simulink model "sistema_completo_discreto_codificado"  (R2023a)
settings: Solver=VariableStepAuto  StartTime=0.0  StopTime=15  MaxStep=1e-3  RelTol=1e-3
values from neighbouring files (symbols this model uses):
  alpha_Cu = 3.9e-3    (= 0.0039)    [variables.m]
  b_a = J_eq * (2*zeta + 1) * omega_pos    [Polos_con_Jeq.m]
  b_eq = b_eq_max    [FrecuenciaNatural_Amortiguamiento.m]    (also in variables.m = 2.19444444444e-05)
  C_ts = 0.818    [variables.m]
  J_eq = J_eq_max    [FrecuenciaNatural_Amortiguamiento.m]    (also in variables.m = 4.58263888889e-05)
  k_l = m*l_cm + m_l*l_l    (= 1)    [variables.m]
  K_sa = J_eq * (2*zeta + 1) * omega_pos^2    [Polos_con_Jeq.m]
  K_sia = J_eq * omega_pos^3    [Polos_con_Jeq.m]
  L_d = 6.6e-3    (= 0.0066)    [variables.m]
  L_ls = 0.8e-3    (= 0.0008)    [variables.m]
  L_q = 5.8e-3    (= 0.0058)    [variables.m]
  lambda_m = 0.016    [variables.m]
  Pp = 3    [variables.m]
  r = 120    [esp_de_operacion.m]    (also in variables.m)
  R_ts = 146.7    [variables.m]
  T_s_ref = 20    [Polos_ceros_Rs.m]
undefined symbols (not defined in the file or in its folder): k_i, k_omega2, k_theta2, omega_n_i, omega_n_pos, omega_n_v, R_s_ref, tau, Ts, Vsl_max, zitta
libraries: SignalEditorBlockLib x5
settings Model: Creator=juanf  LastModifiedBy=Juan

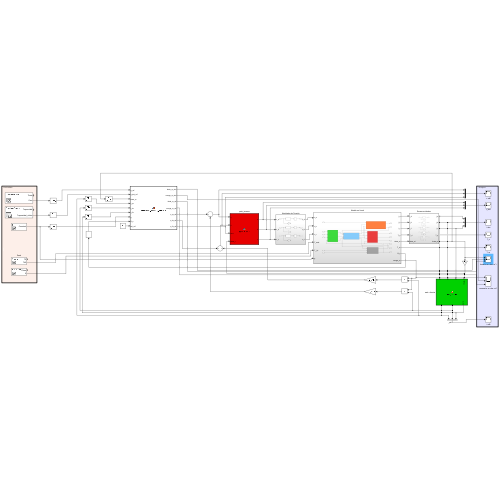
[thumbnail: Simulink's stored preview of the top-level diagram]
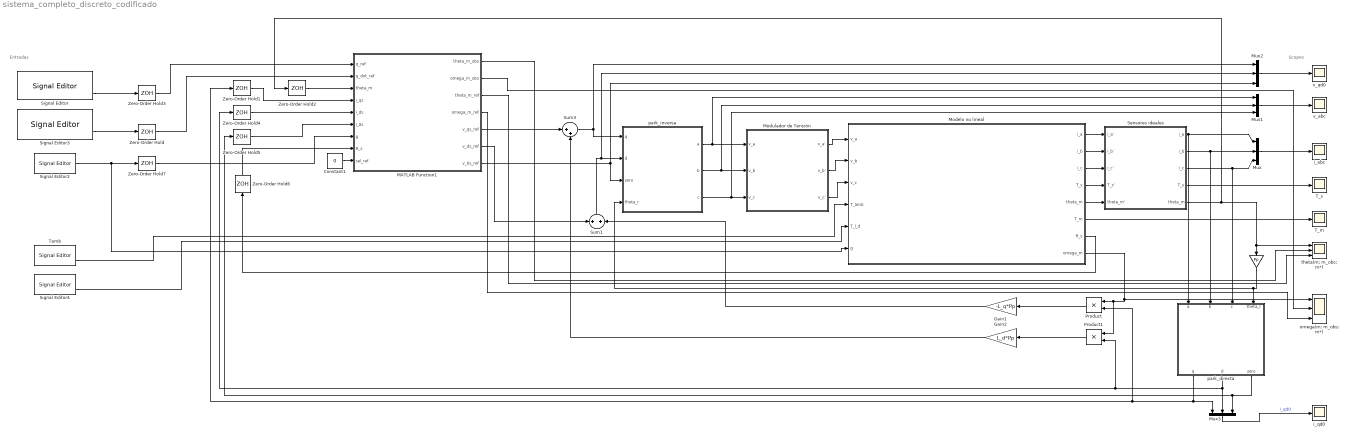
== system sistema_completo_discreto_codificado ==
  note: Scopes
  note: Entradas
  " " : Gain  Gain=Pp
  Constant1 : Constant  Value=0
  Gain1 : Gain  Gain=-L_q*Pp
  Gain2 : Gain  Gain=L_d*Pp
  MATLAB Function1 : MATLAB Function  TreatAsAtomicUnit=on
  Modelo no lineal : Subsystem
  Modulador de Tensión : Subsystem
  Mux{,1..3} (4 alike) : Mux  Inputs=3
  Product : Product
  Product1 : Product
  Sensores ideales : Subsystem
  Signal Editor : SignalEditorBlockLib/Signal Editor  FileName=Consigna_Theta.mat  ActiveScenario=ConsignaTheta  ActiveSignal=Theta  IsBus=off  OutputBusObjectStr=Bus: BusObject  SampleTime=0  ZeroCross=off  OutputAfterFinalValue=Setting to zero  Unit=inherit  PreserveSignalName=on  ApplySigPropsToAllScenarios=on
  Signal Editor2 : SignalEditorBlockLib/Signal Editor  FileName=D:\Facultad\AyME\Automatica-y-maquinas-electricas-final\Matlab - Simulink\señales\g.mat  ActiveScenario=g  ActiveSignal=Constant  IsBus=off  OutputBusObjectStr=Bus: BusObject  SampleTime=0  Interpolate=off  ZeroCross=off  OutputAfterFinalValue=Setting to zero  Unit=inherit  PreserveSignalName=on  ApplySigPropsToAllScenarios=on
  Signal Editor3 : SignalEditorBlockLib/Signal Editor  FileName=D:\Facultad\AyME\Automatica-y-maquinas-electricas-final\Matlab - Simulink\señales\señal_omega_suave.mat  ActiveScenario=ConsignaOmega  ActiveSignal=Trapezoidal  IsBus=off  OutputBusObjectStr=Bus: BusObject  SampleTime=0  Interpolate=off  ZeroCross=off  OutputAfterFinalValue=Setting to zero  Unit=inherit  PreserveSignalName=on  ApplySigPropsToAllScenarios=on
  Signal Editor4 : SignalEditorBlockLib/Signal Editor  FileName=D:\Facultad\AyME\Automatica-y-maquinas-electricas-final\Matlab - Simulink\señales\senal_Tld.mat  ActiveScenario=Senal_Tld  ActiveSignal=Pulse  IsBus=off  OutputBusObjectStr=Bus: BusObject  SampleTime=0  Interpolate=off  ZeroCross=off  OutputAfterFinalValue=Setting to zero  Unit=inherit  PreserveSignalName=on  ApplySigPropsToAllScenarios=on
  Sum1 : Sum  Inputs=+|+
  Sum3 : Sum  Inputs=|++
  T_m : Scope
  T_s : Scope
  Tamb : SignalEditorBlockLib/Signal Editor  FileName=D:\Facultad\AyME\Automatica-y-maquinas-electricas-final\Matlab - Simulink\señales\senal_Tamb.mat  ActiveScenario=T_amb  ActiveSignal=T0  IsBus=off  OutputBusObjectStr=Bus: BusObject  SampleTime=0  Interpolate=off  ZeroCross=off  OutputAfterFinalValue=Setting to zero  Unit=inherit  PreserveSignalName=on  ApplySigPropsToAllScenarios=on
  Zero-Order Hold{,1..7} (8 alike) : ZeroOrderHold  SampleTime=Ts
  i_abc : Scope
  i_qd0 : Scope
  omega(m; m_obs; m*) : Scope  NumInputPorts=3
  park_directa : MATLAB Function  TreatAsAtomicUnit=on
  park_inversa : MATLAB Function  TreatAsAtomicUnit=on
  theta(m; m_obs; m*) : Scope  NumInputPorts=3
  v_abc : Scope
  v_qd0 : Scope
  wires:
  park_inversa/1(a) -> Mux1/1, Modulador de Tensión/1(v_a)
  park_inversa/2(b) -> Mux1/2, Modulador de Tensión/2(v_b)
  park_inversa/3(c) -> Mux1/3, Modulador de Tensión/3(v_c)
  Modulador de Tensión/1(v_a') -> Modelo no lineal/1(v_a)
  Modulador de Tensión/2(v_b') -> Modelo no lineal/2(v_b)
  Modulador de Tensión/3(v_c') -> Modelo no lineal/3(v_c)
  Modelo no lineal/1(i_a) -> Sensores ideales/1(i_a')
  Modelo no lineal/2(i_b) -> Sensores ideales/2(i_b')
  Modelo no lineal/3(i_c) -> Sensores ideales/3(i_c')
  Modelo no lineal/4(T_s) -> Sensores ideales/4(T_s')
  Modelo no lineal/5(theta_m) -> Sensores ideales/5(theta_m')
  Modelo no lineal/6(T_m) -> T_m/1
  Sensores ideales/1(i_a) -> Mux/1, park_directa/1(a)
  Sensores ideales/2(i_b) -> Mux/2, park_directa/2(b)
  Sensores ideales/3(i_c) -> Mux/3, park_directa/3(c)
  Modelo no lineal/8(omega_m) -> Product1/1, Product/1, omega(m; m_obs; m*)/1
  Sum3/1 -> park_inversa/1(q), Mux2/1
  Sensores ideales/4(T_s) -> T_s/1
  park_directa/1(q) -> Product/2, Zero-Order Hold1/1, Mux3/1
  park_directa/2(d) -> Mux3/2, Zero-Order Hold4/1, Product1/2
  park_directa/3(zero) -> Mux3/3, Zero-Order Hold5/1
  " "/1 -> park_inversa/4(theta_r), park_directa/4(theta_r)
  Product/1 -> Gain1/1
  Mux/1 -> i_abc/1
  Mux1/1 -> v_abc/1
  Mux2/1 -> v_qd0/1
  Mux3/1 -> i_qd0/1  "i_qd0"
  Sum1/1 -> Mux2/2, park_inversa/2(d)
  Product1/1 -> Gain2/1
  Gain2/1 -> Sum3/2
  Gain1/1 -> Sum1/2
  Signal Editor2/1 -> Zero-Order Hold7/1, Modelo no lineal/6(g)
  Tamb/2 -> Modelo no lineal/4(T_amb)
  Modelo no lineal/7(R_s) -> Zero-Order Hold6/1
  Signal Editor4/2 -> Modelo no lineal/5(T_l_d)
  Zero-Order Hold/1 -> MATLAB Function1/2(q_dot_ref)
  Zero-Order Hold3/1 -> MATLAB Function1/1(q_ref)
  Signal Editor/2 -> Zero-Order Hold3/1
  Sensores ideales/5(theta_m) -> " "/1, theta(m; m_obs; m*)/1, Zero-Order Hold2/1
  Constant1/1 -> MATLAB Function1/9(sel_ref)
  MATLAB Function1/5(v_qs_ref) -> Sum3/1
  MATLAB Function1/7(v_0s_ref) -> Mux2/3, park_inversa/3(zero)
  MATLAB Function1/6(v_ds_ref) -> Sum1/1
  Zero-Order Hold1/1 -> MATLAB Function1/4(i_qs)
  Zero-Order Hold4/1 -> MATLAB Function1/5(i_ds)
  Zero-Order Hold5/1 -> MATLAB Function1/6(i_0s)
  Zero-Order Hold6/1 -> MATLAB Function1/8(R_s)
  Zero-Order Hold7/1 -> MATLAB Function1/7(g)
  MATLAB Function1/1(theta_m_obs) -> theta(m; m_obs; m*)/2
  MATLAB Function1/3(theta_m_ref) -> theta(m; m_obs; m*)/3
  MATLAB Function1/2(omega_m_obs) -> omega(m; m_obs; m*)/2
  MATLAB Function1/4(omega_m_ref) -> omega(m; m_obs; m*)/3
  Zero-Order Hold2/1 -> MATLAB Function1/3(theta_m)
  Signal Editor3/2 -> Zero-Order Hold/1

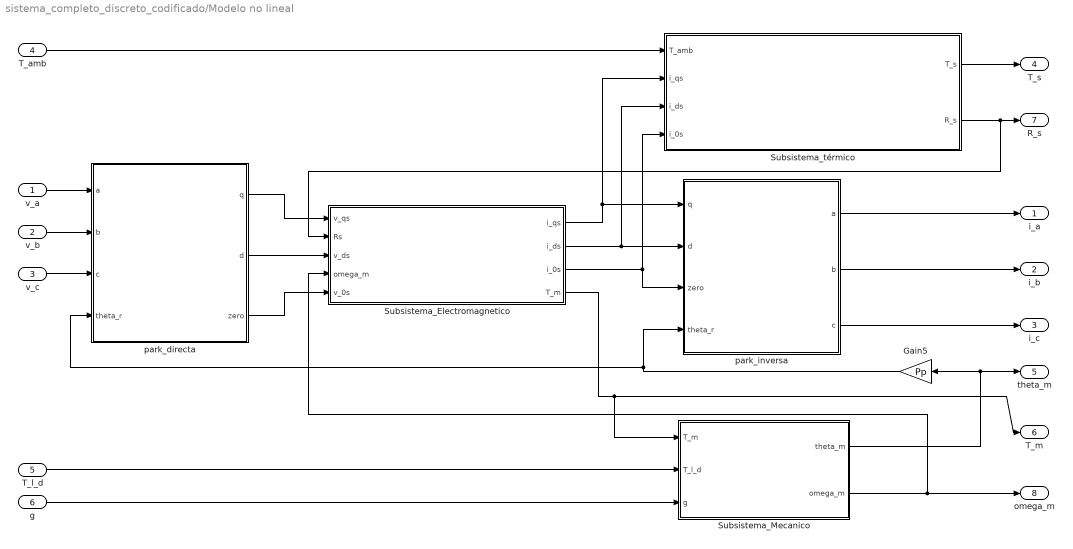
== system sistema_completo_discreto_codificado/Modelo no lineal ==
  v_a : Inport
  v_b : Inport  Port=2
  v_c : Inport  Port=3
  T_amb : Inport  Port=4
  T_l_d : Inport  Port=5
  g : Inport  Port=6
  Gain5 : Gain  Gain=Pp
  Subsistema_Electromagnetico : Subsystem
  Subsistema_Mecanico : Subsystem
  Subsistema_térmico : Subsystem
  park_directa : MATLAB Function  TreatAsAtomicUnit=on
  park_inversa : MATLAB Function  TreatAsAtomicUnit=on
  i_a : Outport
  i_b : Outport  Port=2
  i_c : Outport  Port=3
  T_s : Outport  Port=4
  theta_m : Outport  Port=5
  T_m : Outport  Port=6
  R_s : Outport  Port=7
  omega_m : Outport  Port=8
  wires:
  v_b/1 -> park_directa/2(b)
  Subsistema_Mecanico/1(theta_m) -> theta_m/1, Gain5/1
  T_l_d/1 -> Subsistema_Mecanico/2(T_l_d)
  park_directa/2(d) -> Subsistema_Electromagnetico/3(v_ds)
  Subsistema_Electromagnetico/4(T_m) -> Subsistema_Mecanico/1(T_m), T_m/1
  T_amb/1 -> Subsistema_térmico/1(T_amb)
  Subsistema_térmico/1(T_s) -> T_s/1
  Gain5/1 -> park_directa/4(theta_r), park_inversa/4(theta_r)
  v_a/1 -> park_directa/1(a)
  Subsistema_Mecanico/2(omega_m) -> omega_m/1, Subsistema_Electromagnetico/4(omega_m)
  park_directa/1(q) -> Subsistema_Electromagnetico/1(v_qs)
  Subsistema_térmico/2(R_s) -> Subsistema_Electromagnetico/2(Rs), R_s/1
  v_c/1 -> park_directa/3(c)
  park_inversa/2(b) -> i_b/1
  Subsistema_Electromagnetico/2(i_ds) -> park_inversa/2(d), Subsistema_térmico/3(i_ds)
  park_inversa/1(a) -> i_a/1
  Subsistema_Electromagnetico/1(i_qs) -> park_inversa/1(q), Subsistema_térmico/2(i_qs)
  park_inversa/3(c) -> i_c/1
  Subsistema_Electromagnetico/3(i_0s) -> park_inversa/3(zero), Subsistema_térmico/4(i_0s)
  park_directa/3(zero) -> Subsistema_Electromagnetico/5(v_0s)
  g/1 -> Subsistema_Mecanico/3(g)

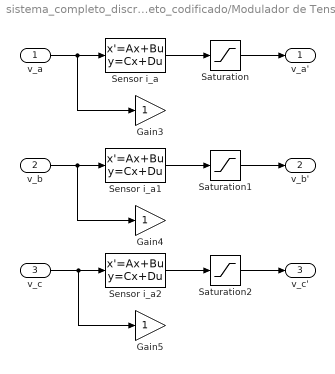
== system sistema_completo_discreto_codificado/Modulador de Tensión ==
  v_a : Inport
  v_b : Inport  Port=2
  v_c : Inport  Port=3
  Gain3 : Gain
  Gain4 : Gain
  Gain5 : Gain
  Saturation : Saturate  UpperLimit=Vsl_max  LowerLimit=-Vsl_max
  Saturation1 : Saturate  UpperLimit=Vsl_max  LowerLimit=-Vsl_max
  Saturation2 : Saturate  UpperLimit=Vsl_max  LowerLimit=-Vsl_max
  Sensor i_a : StateSpace  A=[0 1 ; -omega_n_v^2 -2*zitta*omega_n_v]  B=[0; omega_n_v^2]  C=[1 0]  D=[0]  InitialCondition=0  AllowTunableDMatrix=on
  Sensor i_a1 : StateSpace  A=[0 1 ; -omega_n_v^2 -2*zitta*omega_n_v]  B=[0; omega_n_v^2]  C=[1 0]  D=[0]  InitialCondition=0  AllowTunableDMatrix=on
  Sensor i_a2 : StateSpace  A=[0 1 ; -omega_n_v^2 -2*zitta*omega_n_v]  B=[0; omega_n_v^2]  C=[1 0]  D=[0]  InitialCondition=0  AllowTunableDMatrix=on
  v_a' : Outport
  v_b' : Outport  Port=2
  v_c' : Outport  Port=3
  wires:
  v_b/1 -> Sensor i_a1/1, Gain4/1
  v_a/1 -> Gain3/1, Sensor i_a/1
  Sensor i_a1/1 -> Saturation1/1
  Sensor i_a2/1 -> Saturation2/1
  v_c/1 -> Sensor i_a2/1, Gain5/1
  Sensor i_a/1 -> Saturation/1
  Saturation/1 -> v_a'/1
  Saturation1/1 -> v_b'/1
  Saturation2/1 -> v_c'/1

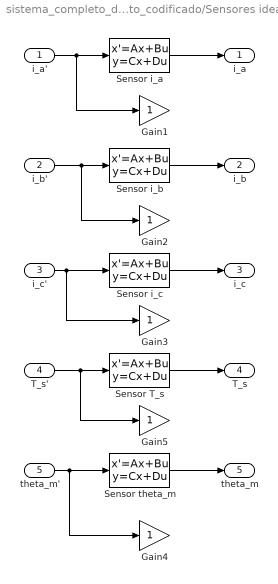
== system sistema_completo_discreto_codificado/Sensores ideales ==
  i_a' : Inport
  i_b' : Inport  Port=2
  i_c' : Inport  Port=3
  T_s' : Inport  Port=4
  theta_m' : Inport  Port=5
  Gain{1..5} (5 alike) : Gain
  Sensor T_s : StateSpace  A=[-1/tau]  B=[1/tau]  C=[1]  D=[0]  InitialCondition=40  AllowTunableDMatrix=on
  Sensor i_a : StateSpace  A=[0 1 ; -omega_n_i^2 -2*zitta*omega_n_i]  B=[0; omega_n_i^2]  C=[1 0]  D=[0]  InitialCondition=0  AllowTunableDMatrix=on
  Sensor i_b : StateSpace  A=[0 1 ; -omega_n_i^2 -2*zitta*omega_n_i]  B=[0; omega_n_i^2]  C=[1 0]  D=[0]  InitialCondition=0  AllowTunableDMatrix=on
  Sensor i_c : StateSpace  A=[0 1 ; -omega_n_i^2 -2*zitta*omega_n_i]  B=[0; omega_n_i^2]  C=[1 0]  D=[0]  InitialCondition=0  AllowTunableDMatrix=on
  Sensor theta_m : StateSpace  A=[0 1 ; -omega_n_pos^2 -2*zitta*omega_n_pos]  B=[0; omega_n_pos^2]  C=[1 0]  D=[0]  InitialCondition=0  AllowTunableDMatrix=on
  i_a : Outport
  i_b : Outport  Port=2
  i_c : Outport  Port=3
  T_s : Outport  Port=4
  theta_m : Outport  Port=5
  wires:
  i_a'/1 -> Gain1/1, Sensor i_a/1
  i_b'/1 -> Gain2/1, Sensor i_b/1
  i_c'/1 -> Gain3/1, Sensor i_c/1
  T_s'/1 -> Gain5/1, Sensor T_s/1
  theta_m'/1 -> Gain4/1, Sensor theta_m/1
  Sensor theta_m/1 -> theta_m/1
  Sensor T_s/1 -> T_s/1
  Sensor i_c/1 -> i_c/1
  Sensor i_b/1 -> i_b/1
  Sensor i_a/1 -> i_a/1

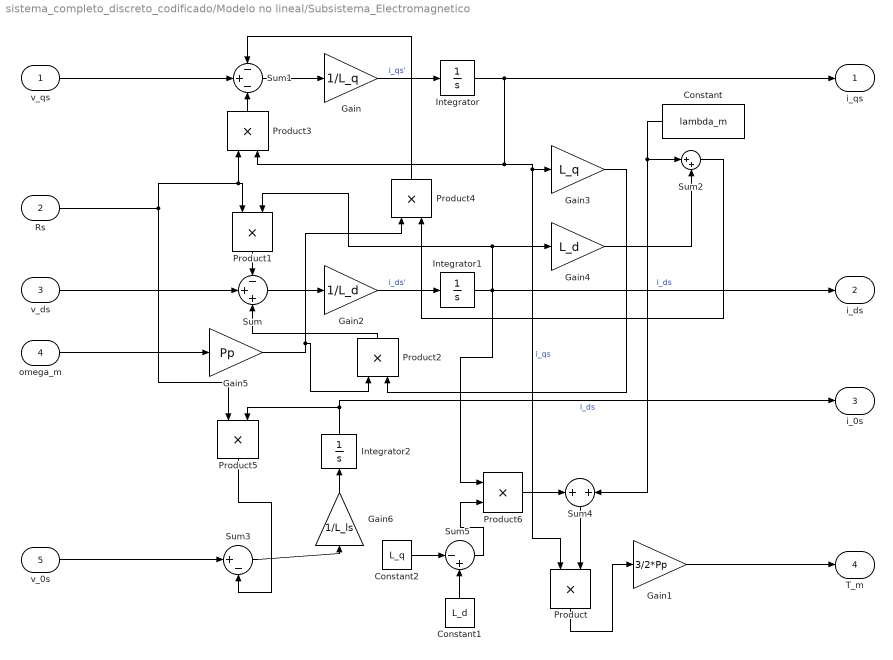
== system sistema_completo_discreto_codificado/Modelo no lineal/Subsistema_Electromagnetico ==
  v_qs : Inport
  Rs : Inport  Port=2
  v_ds : Inport  Port=3
  omega_m : Inport  Port=4
  v_0s : Inport  Port=5
  Constant : Constant  Value=lambda_m
  Constant1 : Constant  Value=L_d
  Constant2 : Constant  Value=L_q
  Gain : Gain  Gain=1/L_q
  Gain1 : Gain  Gain=3/2*Pp
  Gain2 : Gain  Gain=1/L_d
  Gain3 : Gain  Gain=L_q
  Gain4 : Gain  Gain=L_d
  Gain5 : Gain  Gain=Pp
  Gain6 : Gain  Gain=1/L_ls
  Integrator : Integrator
  Integrator1 : Integrator
  Integrator2 : Integrator
  Product{,1..6} (7 alike) : Product
  Sum : Sum  Inputs=-++
  Sum1 : Sum  Inputs=-+-
  Sum2 : Sum  Inputs=|++
  Sum3 : Sum  Inputs=|+-
  Sum4 : Sum
  Sum5 : Sum  Inputs=|-+
  i_qs : Outport
  i_ds : Outport  Port=2
  i_0s : Outport  Port=3
  T_m : Outport  Port=4
  wires:
  Gain1/1 -> T_m/1
  Product/1 -> Gain1/1
  v_qs/1 -> Sum1/2
  Sum1/1 -> Gain/1
  Gain/1 -> Integrator/1  "i_qs'"
  Integrator/1 -> Product/1, Gain3/1, Product3/2, i_qs/1  "i_qs"
  Product3/1 -> Sum1/3
  Rs/1 -> Product3/1, Product1/1, Product5/1
  Product4/1 -> Sum1/1
  Product1/1 -> Sum/1
  v_ds/1 -> Sum/2
  Sum/1 -> Gain2/1
  Gain2/1 -> Integrator1/1  "i_ds'"
  Integrator1/1 -> i_ds/1, Product6/1, Gain4/1, Product1/2  "i_ds"
  Constant/1 -> Sum4/2, Sum2/1
  Sum2/1 -> Product4/2
  omega_m/1 -> Gain5/1
  Gain5/1 -> Product2/1, Product4/1
  Product2/1 -> Sum/3
  Gain4/1 -> Sum2/2
  Gain3/1 -> Product2/2
  v_0s/1 -> Sum3/1
  Product5/1 -> Sum3/2
  Sum3/1 -> Gain6/1
  Gain6/1 -> Integrator2/1
  Integrator2/1 -> Product5/2, i_0s/1  "i_ds"
  Constant1/1 -> Sum5/2
  Constant2/1 -> Sum5/1
  Product6/1 -> Sum4/1
  Sum5/1 -> Product6/2
  Sum4/1 -> Product/2

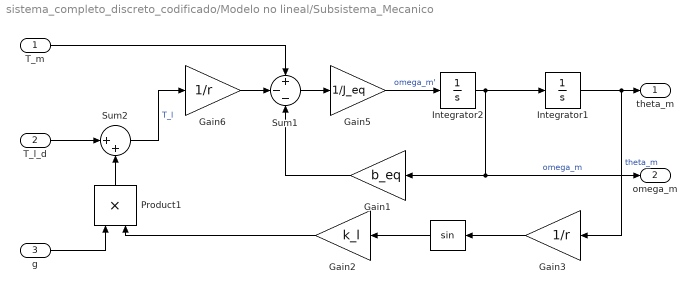
== system sistema_completo_discreto_codificado/Modelo no lineal/Subsistema_Mecanico ==
  T_m : Inport
  T_l_d : Inport  Port=2
  g : Inport  Port=3
  " " : Trigonometry
  Gain1 : Gain  Gain=b_eq
  Gain2 : Gain  Gain=k_l
  Gain3 : Gain  Gain=1/r
  Gain5 : Gain  Gain=1/J_eq
  Gain6 : Gain  Gain=1/r
  Integrator1 : Integrator
  Integrator2 : Integrator
  Product1 : Product
  Sum1 : Sum  Inputs=+--
  Sum2 : Sum  Inputs=|++
  theta_m : Outport
  omega_m : Outport  Port=2
  wires:
  Product1/1 -> Sum2/2
  T_l_d/1 -> Sum2/1
  Integrator1/1 -> Gain3/1, theta_m/1  "theta_m"
  Gain3/1 -> " "/1
  " "/1 -> Gain2/1
  Gain1/1 -> Sum1/3
  Sum1/1 -> Gain5/1
  Sum2/1 -> Gain6/1  "T_l"
  Gain6/1 -> Sum1/2
  Integrator2/1 -> Integrator1/1, Gain1/1, omega_m/1  "omega_m"
  Gain5/1 -> Integrator2/1  "omega_m'"
  Gain2/1 -> Product1/2
  T_m/1 -> Sum1/1
  g/1 -> Product1/1

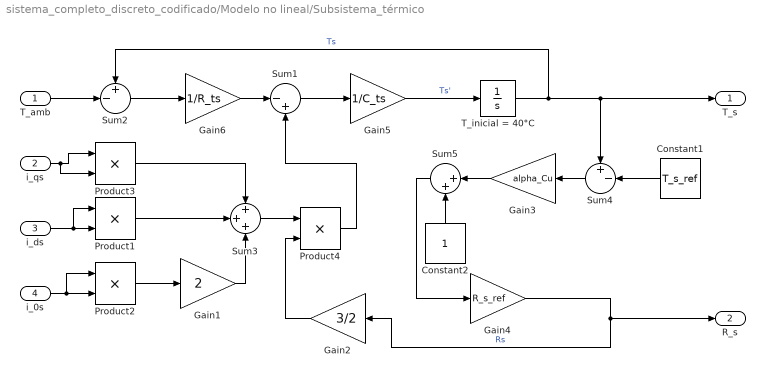
== system sistema_completo_discreto_codificado/Modelo no lineal/Subsistema_térmico ==
  T_amb : Inport
  i_qs : Inport  Port=2
  i_ds : Inport  Port=3
  i_0s : Inport  Port=4
  Constant1 : Constant  Value=T_s_ref
  Constant2 : Constant
  Gain1 : Gain  Gain=2
  Gain2 : Gain  Gain=3/2
  Gain3 : Gain  Gain=alpha_Cu
  Gain4 : Gain  Gain=R_s_ref
  Gain5 : Gain  Gain=1/C_ts
  Gain6 : Gain  Gain=1/R_ts
  Product{1..4} (4 alike) : Product
  Sum1 : Sum  Inputs=|-+
  Sum2 : Sum  Inputs=+-|
  Sum3 : Sum  Inputs=+++
  Sum4 : Sum  Inputs=+-|
  Sum5 : Sum  Inputs=|++
  T_inicial = 40°C : Integrator  InitialCondition=40
  T_s : Outport
  R_s : Outport  Port=2
  wires:
  Gain5/1 -> T_inicial = 40°C/1  "Ts'"
  Sum1/1 -> Gain5/1
  Sum2/1 -> Gain6/1
  T_amb/1 -> Sum2/2
  T_inicial = 40°C/1 -> Sum4/1, T_s/1, Sum2/1  "Ts"
  i_qs/1 -> Product3/2, Product3/1
  i_0s/1 -> Product2/1, Product2/2
  Product2/1 -> Gain1/1
  Gain1/1 -> Sum3/3
  Product1/1 -> Sum3/2
  Product3/1 -> Sum3/1
  Sum3/1 -> Product4/1
  Gain2/1 -> Product4/2
  Gain6/1 -> Sum1/1
  Product4/1 -> Sum1/2
  Constant1/1 -> Sum4/2
  Sum4/1 -> Gain3/1
  Constant2/1 -> Sum5/2
  Sum5/1 -> Gain4/1
  Gain4/1 -> Gain2/1, R_s/1  "Rs"
  Gain3/1 -> Sum5/1
  i_ds/1 -> Product1/2, Product1/1

== matlab function sistema_completo_discreto_codificado/MATLAB Function1 ==
  data: q_ref input; q_dot_ref input; theta_m input; i_qs input; i_ds input; i_0s input; g input; R_s input; Ts parameter; r parameter; J_eq parameter; b_a parameter; K_sa parameter; K_sia parameter; k_i parameter; k_theta2 parameter; theta_m_obs output; omega_m_obs output; k_omega2 parameter; b_eq parameter; k_l parameter; Pp parameter; lambda_m parameter; L_d parameter; L_q parameter; L_ls parameter; theta_m_ref output; omega_m_ref output; sel_ref input; v_qs_ref output; v_ds_ref output; v_0s_ref output
function [theta_m_obs, omega_m_obs, theta_m_ref, omega_m_ref, ...
          v_qs_ref, v_ds_ref, v_0s_ref] = controlador_discreto_completo( ...
          q_ref, q_dot_ref, theta_m, i_qs, i_ds, i_0s, g, R_s, ...
          Ts, r, J_eq, b_a, K_sa, K_sia, k_i, k_theta2, k_omega2, ...
          b_eq, k_l, Pp, lambda_m, L_d, L_q, L_ls, sel_ref)
%CONTROLADOR_DISCRETO_COMPLETO
% Reemplaza en una sola MATLAB Function todos los bloques externos a la
% planta del modelo discreto:
%   1) Setpoint
%   2) PID externo
%   3) Observador
%   4) Modulador de torque
%   5) Modulador de corriente
%   6) Desacople electromagnetico
%
% Para que reemplace tambien a los Zero-Order Hold del esquema, el bloque
% MATLAB Function debe ejecutarse con tiempo de muestreo Ts.

persistent initialized

persistent C_halfTs C_invJeq C_invTs
persistent C_r C_inv_r
persistent C_ba C_Ksa C_Ksia
persistent C_ktheta2 C_komega2 C_ki
persistent C_beq C_kg_over_r C_three_halves_pp
persistent C_lambda_m C_Ld C_Lq C_Lls
persistent C_Ld_minus_Lq
persistent C_kiq C_kid C_ki0

% Memorias para generacion de referencias
persistent ref_theta_prev
persistent ref_omega_u_prev ref_omega_y_prev

% PID externo
persistent pid_u1_prev pid_y1_prev
persistent pid_u2_prev pid_y2_prev

% Observador
persistent obs_z_eps obs_z_alpha obs_z_thetadot
persistent obs_xi_u_prev obs_xi_y_prev
persistent obs_omega_u_prev obs_omega_y_prev
persistent obs_theta_u_prev obs_theta_y_prev

if isempty(initialized)
    initialized = true;

    C_halfTs = Ts / 2;
    C_invJeq = 1 / J_eq;
    C_invTs  = 1 / Ts;

    C_r     = r;
    C_inv_r = 1 / r;

    C_ba    = b_a;
    C_Ksa   = K_sa;
    C_Ksia  = K_sia;

    C_ktheta2 = k_theta2;
    C_komega2 = k_omega2;
    C_ki      = k_i;

    C_beq             = b_eq;
    C_kg_over_r       = k_l / r;
    C_three_halves_pp = 1.5 * Pp;

    C_lambda_m    = lambda_m;
    C_Ld          = L_d;
    C_Lq          = L_q;
    C_Lls         = L_ls;
    C_Ld_minus_Lq = L_d - L_q;

    C_kiq = 5000 * L_q;
    C_kid = 5000 * L_d;
    C_ki0 = 5000 * L_ls;

    ref_theta_prev   = 0;
    ref_omega_u_prev = 0;
    ref_omega_y_prev = 0;

    pid_u1_prev = 0;
    pid_y1_prev = 0;
    pid_u2_prev = 0;
    pid_y2_prev = 0;

    obs_z_eps      = 0;
    obs_z_alpha    = 0;
    obs_z_thetadot = 0;

    obs_xi_u_prev    = 0;
    obs_xi_y_prev    = 0;
    obs_omega_u_prev = 0;
    obs_omega_y_prev = 0;
    obs_theta_u_prev = 0;
    obs_theta_y_prev = 0;
end

% =========================================================================
% A) OBSERVADOR: SALIDAS ESTIMADAS
% =========================================================================
[x_I, obs_xi_u_prev, obs_xi_y_prev] = ...
    f_tustin(obs_z_eps, obs_xi_u_prev, obs_xi_y_prev, C_halfTs);

[omega_m_obs, obs_omega_u_prev, obs_omega_y_prev] = ...
    f_tustin(obs_z_alpha, obs_omega_u_prev, obs_omega_y_prev, C_halfTs);

[theta_m_obs, obs_theta_u_prev, obs_theta_y_prev] = ...
    f_tustin(obs_z_thetadot, obs_theta_u_prev, obs_theta_y_prev, C_halfTs);

% =========================================================================
% B) GENERACION DE REFERENCIAS
% sel_ref = 0 -> referencia principal de velocidad
% sel_ref = 1 -> referencia principal de posicion
% =========================================================================
if sel_ref == 0
    omega_m_ref = C_r * q_dot_ref;

    [theta_m_ref, ref_omega_u_prev, ref_omega_y_prev] = ...
        f_tustin(omega_m_ref, ref_omega_u_prev, ref_omega_y_prev, C_halfTs);

    ref_theta_prev = theta_m_ref;
else
    theta_m_ref = C_r * q_ref;
    omega_m_ref = (theta_m_ref - ref_theta_prev) * C_invTs;

    ref_theta_prev = theta_m_ref;

    ref_omega_u_prev = omega_m_ref;
    ref_omega_y_prev = theta_m_ref;
end

% =========================================================================
% C) CONTROLADOR EXTERNO
% =========================================================================
e_omega = omega_m_ref - omega_m_obs;

[p_k, pid_u1_prev, pid_y1_prev] = ...
    f_tustin(e_omega, pid_u1_prev, pid_y1_prev, C_halfTs);

[I_k, pid_u2_prev, pid_y2_prev] = ...
    f_tustin(p_k, pid_u2_prev, pid_y2_prev, C_halfTs);

T_m_ref = C_ba * e_omega + C_Ksa * p_k + C_Ksia * I_k;

% =========================================================================
% D) ACTUALIZACION DEL OBSERVADOR
% =========================================================================
eps_k      = theta_m - theta_m_obs;
alpha_k    = T_m_ref * C_invJeq + C_komega2 * eps_k + C_ki * x_I;
thetadot_k = omega_m_obs + C_ktheta2 * eps_k;

obs_z_eps      = eps_k;
obs_z_alpha    = alpha_k;
obs_z_thetadot = thetadot_k;

% =========================================================================
% E) MODULADOR DE TORQUE
% =========================================================================
i_ds_ref = 0;
i_0s_ref = 0;

torque_num = C_kg_over_r * g * sin(C_inv_r * theta_m_obs) ...
           + T_m_ref ...
           + C_beq * omega_m_obs;

torque_den = C_three_halves_pp * ...
           (C_Ld_minus_Lq * i_ds + C_lambda_m);

i_qs_ref = torque_num / torque_den;

% =========================================================================
% F) MODULADOR DE CORRIENTE
% =========================================================================
v_qs_pi = C_kiq * (i_qs_ref - i_qs);
v_ds_pi = C_kid * (i_ds_ref - i_ds);
v_0s_pi = C_ki0 * (i_0s_ref - i_0s);

% =========================================================================
% G) DESACOPLE ELECTROMAGNETICO
% =========================================================================
omega_e = Pp * omega_m_obs;

v_qs_ref = v_qs_pi ...
         + omega_e * (C_Ld * i_ds + C_lambda_m) ...
         + R_s * i_qs;

v_ds_ref = v_ds_pi ...
         - omega_e * C_Lq * i_qs ...
         + R_s * i_ds;

v_0s_ref = v_0s_pi + R_s * i_0s;

end


function [y, u_prev, y_prev] = f_tustin(u, u_prev, y_prev, half_Ts)
    y = y_prev + half_Ts * (u + u_prev);
    u_prev = u;
    y_prev = y;
end

== matlab function sistema_completo_discreto_codificado/park_inversa ==
  data: q input; a output; d input; zero input; theta_r input; b output; c output
function [a, b, c] = park_inversa(q, d, zero, theta_r)
% qd0 → abc (transformacion inversa)
% Entradas: q, d, zero (coordenadas qd0), theta_r (ángulo eléctrico)
% Salidas: a, b, c (señales de fase)
    
    T_inv = [cos(theta_r),               sin(theta_r),              1;
             cos(theta_r - 2*pi/3),      sin(theta_r - 2*pi/3),     1;
             cos(theta_r + 2*pi/3),      sin(theta_r + 2*pi/3),     1];
    
    abc = T_inv * [q; d; zero];

    a = abc(1);
    b = abc(2);
    c = abc(3);
end

== matlab function sistema_completo_discreto_codificado/park_directa ==
  data: a input; q output; b input; c input; theta_r input; d output; zero output
function [q, d, zero] = park_directa(a, b, c, theta_r)
% Transformacion abc → qd0
% a, b y c son señales de fase y theta_r es el angulo ELECTRICO (no mecanico) del rotor)
% Salidas: q, d, zero, que son las coordenadas virtuales qd0
    
    T = (2/3) * [cos(theta_r),           cos(theta_r - 2*pi/3),      cos(theta_r + 2*pi/3);
                 sin(theta_r),           sin(theta_r - 2*pi/3),      sin(theta_r + 2*pi/3);
                 1/2,                    1/2,                         1/2];
    
    qd0 = T * [a; b; c];
    
% asignar salidas
    q = qd0(1);
    d = qd0(2);
    zero = qd0(3);
end

== matlab function sistema_completo_discreto_codificado/Modelo no lineal/park_directa ==
  data: a input; q output; b input; c input; theta_r input; d output; zero output
function [q, d, zero] = park_directa(a, b, c, theta_r)
% Transformacion abc → qd0
% a, b y c son señales de fase y theta_r es el angulo ELECTRICO (no mecanico) del rotor)
% Salidas: q, d, zero, que son las coordenadas virtuales qd0
    
    T = (2/3) * [cos(theta_r),           cos(theta_r - 2*pi/3),      cos(theta_r + 2*pi/3);
                 sin(theta_r),           sin(theta_r - 2*pi/3),      sin(theta_r + 2*pi/3);
                 1/2,                    1/2,                         1/2];
    
    qd0 = T * [a; b; c];
    
% asignar salidas
    q = qd0(1);
    d = qd0(2);
    zero = qd0(3);
end

== matlab function sistema_completo_discreto_codificado/Modelo no lineal/park_inversa ==
  data: q input; a output; d input; zero input; theta_r input; b output; c output
function [a, b, c] = park_inversa(q, d, zero, theta_r)
% qd0 → abc (transformacion inversa)
% Entradas: q, d, zero (coordenadas qd0), theta_r (ángulo eléctrico)
% Salidas: a, b, c (señales de fase)
    
    T_inv = [cos(theta_r),               sin(theta_r),              1;
             cos(theta_r - 2*pi/3),      sin(theta_r - 2*pi/3),     1;
             cos(theta_r + 2*pi/3),      sin(theta_r + 2*pi/3),     1];
    
    abc = T_inv * [q; d; zero];

    a = abc(1);
    b = abc(2);
    c = abc(3);
end
